simulink model "nxt2nxt"  (Simulink 6.4)
settings: Solver=FixedStepDiscrete  StartTime=0.0  StopTime=inf  FixedStep=0.001  RelTol=1e-3
undefined symbols (not defined in the file): clearNXTSignalObjects
libraries: simulink x2
settings Model: LastModifiedBy=takashic  ProdHWDeviceType=ARM7
settings DataIOCC: LimitDataPoints=off  SaveOutput=off  SignalLogging=off  SaveTime=off
settings OptimizationCC: InlineParams=on  InlineInvariantSignals=on  EnforceIntegerDowncast=off  StateBitsets=on  DataBitsets=on  UseTempVars=on  ZeroExternalMemoryAtStartup=off  ZeroInternalMemoryAtStartup=off  NoFixptDivByZeroProtection=on  EfficientFloat2IntCast=on  OptimizeModelRefInitCode=on  LifeSpan=1
settings DebuggingCC: ReadBeforeWriteMsg=DisableAll  WriteAfterWriteMsg=DisableAll  WriteAfterReadMsg=DisableAll  MultiTaskDSMMsg=none  ParameterDowncastMsg=warning  ParameterOverflowMsg=warning  ParameterUnderflowMsg=warning
settings HardwareCC: ProdIntDivRoundTo=Zero  ProdEndianess=LittleEndian  ProdHWDeviceType=ARM7
settings RTWCC: SystemTargetFile=ert.tlc  GenCodeOnly=on  TemplateMakefile=ert_default_tmf  Description=Real-Time Workshop Embedded Coder (no auto configuration)  RTWVerbose=off  ProcessScript=ert_make_rtw_hook
settings CodeAppCC: IgnoreCustomStorageClasses=off
settings ERTTargetCC: TargetFcnLib=ansi_tfl_tmw.mat  GenFloatMathFcnCalls=ANSI_C  IncludeMdlTerminateFcn=off  SuppressErrorStatus=on  IncludeERTFirstTime=on  SupportAbsoluteTime=off  SupportNonFinite=off  SupportComplex=off  InlinedParameterPlacement=NonHierarchical  ERTCustomFileTemplate=example_file_process.tlc  InitialValueSource=Model

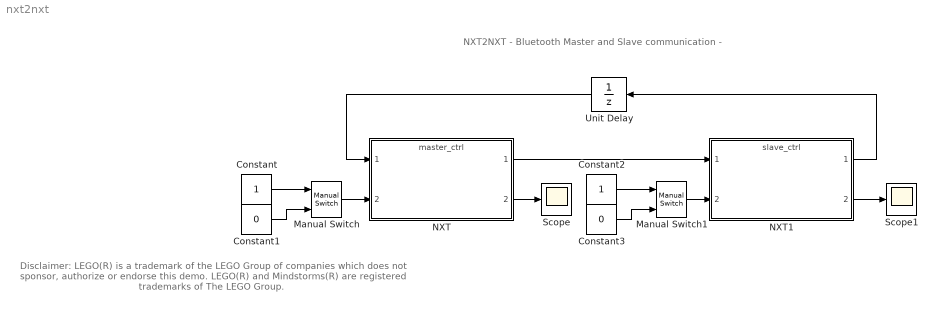
== system nxt2nxt ==
  note: NXT2NXT - Bluetooth Master and Slave communication -
  note: Disclaimer:
      | LEGO(R) is a trademark of the LEGO Group of companies which does not sponsor, authorize or endorse this demo.
      | LEGO(R) and Mindstorms(R)  are registered trademarks of The LEGO Group.
  Constant : Constant  Value=1  OutDataTypeMode=uint8  OutDataType=sfix(16)  ConRadixGroup=Use specified scaling  OutScaling=2^0  SampleTime=inf  FramePeriod=inf
  Constant1 : Constant  Value=0  OutDataTypeMode=uint8  OutDataType=sfix(16)  ConRadixGroup=Use specified scaling  OutScaling=2^0  SampleTime=inf  FramePeriod=inf
  Constant2 : Constant  Value=1  OutDataTypeMode=uint8  OutDataType=sfix(16)  ConRadixGroup=Use specified scaling  OutScaling=2^0  SampleTime=inf  FramePeriod=inf
  Constant3 : Constant  Value=0  OutDataTypeMode=uint8  OutDataType=sfix(16)  ConRadixGroup=Use specified scaling  OutScaling=2^0  SampleTime=inf  FramePeriod=inf
  Manual Switch : simulink/Signal Routing/Manual Switch  SystemSampleTime=-1  sw=0  action=0
  Manual Switch1 : simulink/Signal Routing/Manual Switch  SystemSampleTime=-1  sw=0  action=0
  NXT : ModelReference  StartFcn=%clearNXTSignalObjects();  ModelName=master_ctrl  ModelReferenceVersion=1.192  CopyOfModelName=master_ctrl
      mask init:
      | [data, map]=imread('NXT_ICON.gif');
      | pic=ind2rgb(data,map);
      mask Display: image(pic,  [45, 8, 50, 50])
  NXT1 : ModelReference  StartFcn=%clearNXTSignalObjects();  ModelName=slave_ctrl  ModelReferenceVersion=1.187  CopyOfModelName=slave_ctrl
      mask init:
      | [data, map]=imread('NXT_ICON.gif');
      | pic=ind2rgb(data,map);
      mask Display: image(pic,  [45, 8, 50, 50])
  Scope : Scope
      settings: TimeRange=400  YMax=105
  Scope1 : Scope
      settings: TimeRange=400  YMax=105
  Unit Delay : UnitDelay  Orientation=left  SampleTime=-1
  wires:
  NXT/1 -> NXT1/1
  NXT1/1 -> Unit Delay/1
  Manual Switch/1 -> NXT/2
  Constant/1 -> Manual Switch/1
  Constant1/1 -> Manual Switch/2
  Constant2/1 -> Manual Switch1/1
  Constant3/1 -> Manual Switch1/2
  Manual Switch1/1 -> NXT1/2
  NXT/2 -> Scope/1
  NXT1/2 -> Scope1/1
  Unit Delay/1 -> NXT/1
